simulink model "Neurofeedback_PID_WithoutFNIRS"  (R2021b)
settings: Solver=VariableStepAuto  StartTime=0.0  StopTime=90  FixedStep=0.09  RelTol=1e-8
libraries: slpidlib x1
settings Model: SnapshotInterval=100  Creator=mdls3  LastModifiedBy=mdls3
settings SolverCC: ZeroCrossControl=EnableAll
settings DebuggingCC: UnderSpecifiedDimensionMsg=warning

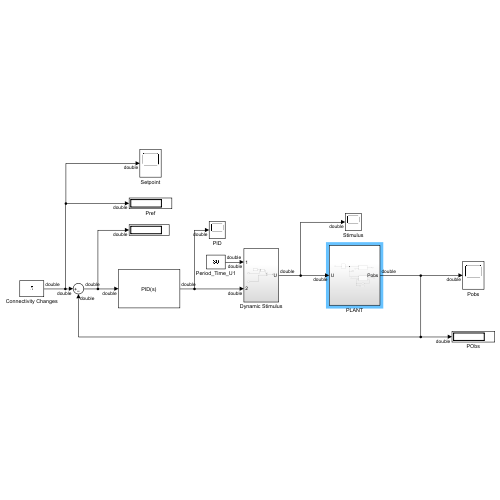
[thumbnail: Simulink's stored preview of the top-level diagram]
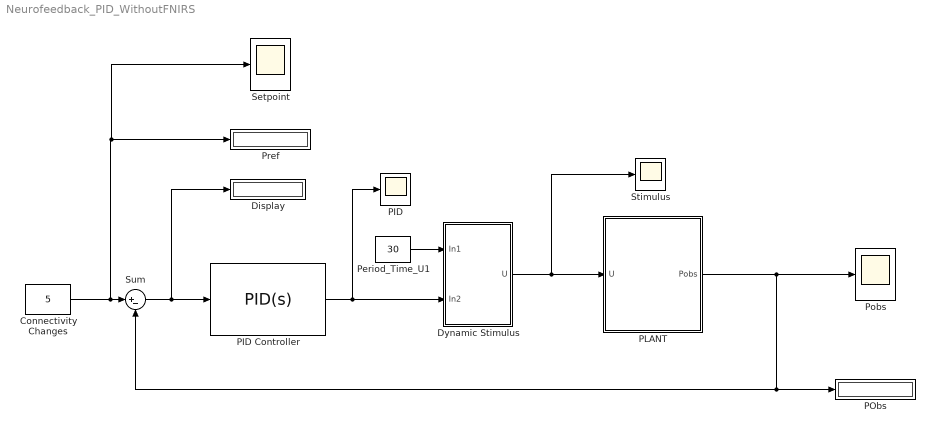
== system Neurofeedback_PID_WithoutFNIRS ==
  Connectivity Changes : Constant  Value=5
  Display : Display
  Dynamic Stimulus : Subsystem
  PID : Scope
  PID Controller : slpidlib/PID Controller  Controller=PID  Form=Ideal  TimeDomain=Continuous-time  UseExternalTs=off  SampleTime=-1  IntegratorMethod=Forward Euler  FilterMethod=Forward Euler  ControllerParametersSource=internal  P=0.2  I=0.1525  D=0.105  UseFilter=on  N=100  TunerSelectOption=Transfer Function Based (PID Tuner App)  InitialConditionSource=internal  InitialConditionForIntegrator=1  InitialConditionForFilter=0  DifferentiatorICPrevScaledInput=0  ExternalReset=none  TrackingMode=off  Kt=1  LimitOutput=off  SatLimitsSource=internal  UpperSaturationLimit=inf  LowerSaturationLimit=-inf  LinearizeAsGain=on  AntiWindupMode=none  Kb=1  POutMin=[]  POutMax=[]  IOutMin=[]  IOutMax=[]  DOutMin=[]  DOutMax=[]  NOutMin=[]  NOutMax=[]  SumOutMin=[]  SumOutMax=[]  SaturationOutMin=[]  SaturationOutMax=[]  PParamMin=[]  PParamMax=[]  IParamMin=[]  IParamMax=[]  DParamMin=[]  DParamMax=[]  NParamMin=[]  NParamMax=[]  KbParamMin=[]  KbParamMax=[]  KtParamMin=[]  KtParamMax=[]  KbOutMin=[]  KbOutMax=[]  KtOutMin=[]  KtOutMax=[]  IntegratorOutMin=[]  IntegratorOutMax=[]  FilterOutMin=[]  FilterOutMax=[]  SumI1OutMin=[]  SumI1OutMax=[]  SumI2OutMin=[]  SumI2OutMax=[]  SumI3OutMin=[]  SumI3OutMax=[]  SumI4OutMin=[]  SumI4OutMax=[]  SumDOutMin=[]  SumDOutMax=[]  DifferentiatorOutMin=[]  DifferentiatorOutMax=[]  FilterDiffOutCoefMin=[]  FilterDiffOutCoefMax=[]  ReciprocalOutMin=[]  ReciprocalOutMax=[]  SumDenOutMin=[]  SumDenOutMax=[]  SumNumOutMin=[]  SumNumOutMax=[]  DivideOutMin=[]  DivideOutMax=[]  UdiffTsProdOutMin=[]  UdiffTsProdOutMax=[]  NTsProdOutMin=[]  NTsProdOutMax=[]  UintegralTsProdOutMin=[]  UintegralTsProdOutMax=[]  UngainTsProdOutMin=[]  UngainTsProdOutMax=[]  IntegratorContinuousStateAttributes=''  IntegratorStateMustResolveToSignalObject=off  IntegratorRTWStateStorageClass=Auto  FilterContinuousStateAttributes=''  FilterStateMustResolveToSignalObject=off  FilterRTWStateStorageClass=Auto  ParallelPVariant=Passthrough  IdealPVariant=InternalParameters  IVariant=InternalParameters  DVariant=InternalParameters  IntegratorVariant=Continuous  SatVariant=Disabled  AWVariant=Passthrough  PCopyVariant=Disabled  TRVariant=Disabled  FdbkBlocksVariant=Forward  IdealPFdbkVariant=Disabled  SatFdbkVariant=Disabled  DerivativeFilterVariant=ContFilter  NVariant=InternalParameters  NCopyVariant=Disabled  FilterICVariant=InternalICsFilter  IntegratorICVariant=InternalICs  ExternalResetVariant=Disabled  TRSumVariant=Passthrough  SumFdbkVariant=Disabled  SumVariant=Sum_PID  TsampFilterVariant=InternalTs  TsampNgainVariant=Passthrough  TsampIntegralVariant=Passthrough  ExternalSaturationOutDataTypeStr=Inherit: Same as second input
  PLANT : Subsystem
  PObs : Display
  Period_Time_U1 : Constant  Value=30
  Pobs : Scope
  Pref : Display
  Setpoint : Scope
  Stimulus : Scope
  Sum : Sum  Inputs=|+-
  wires:
  Period_Time_U1/1 -> Dynamic Stimulus/1(In1)
  Dynamic Stimulus/1(U) -> Stimulus/1, PLANT/1(U)
  PID Controller/1 -> Dynamic Stimulus/2(In2), PID/1
  Sum/1 -> PID Controller/1, Display/1
  Connectivity Changes/1 -> Setpoint/1, Pref/1, Sum/1
  PLANT/1(Pobs) -> Sum/2, PObs/1, Pobs/1

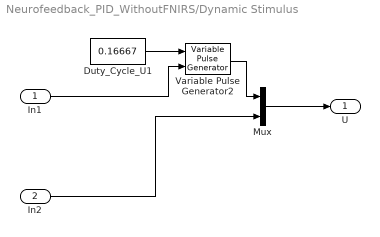
== system Neurofeedback_PID_WithoutFNIRS/Dynamic Stimulus ==
  In1 : Inport
  In2 : Inport  Port=2
  Duty_Cycle_U1 : Constant  Value=0.16667  OutMin=[0]  OutMax=[0.8]
  Mux : Mux  Inputs=2
  Variable Pulse Generator2 : VariablePulseGenerator  RunAtFixedTimeIntervals=on  SampleTime=1/10.4
  U : Outport
  wires:
  In1/1 -> Variable Pulse Generator2/2
  Mux/1 -> U/1
  Variable Pulse Generator2/1 -> Mux/1
  Duty_Cycle_U1/1 -> Variable Pulse Generator2/1
  In2/1 -> Mux/2

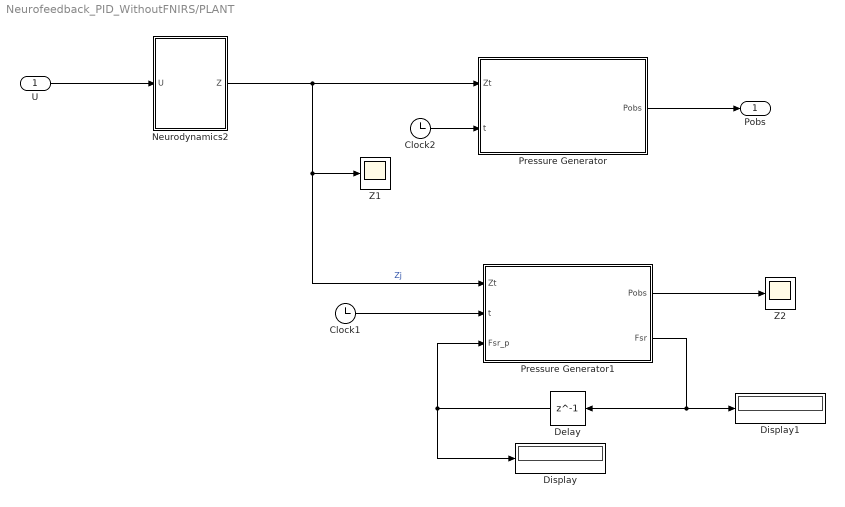
== system Neurofeedback_PID_WithoutFNIRS/PLANT ==
  U : Inport
  Clock1 : Clock
  Clock2 : Clock
  Delay : Delay  DelayLength=1  InitialCondition=0.0001
  Display : Display
  Display1 : Display
  Neurodynamics2 : Subsystem
  Pressure Generator : MATLAB Function  TreatAsAtomicUnit=on
  Pressure Generator1 : MATLAB Function  TreatAsAtomicUnit=on
  Z1 : Scope
  Z2 : Scope
  Pobs : Outport
  wires:
  U/1 -> Neurodynamics2/1(U)
  Neurodynamics2/1(Z) -> Pressure Generator/1(Zt), Pressure Generator1/1(Zt), Z1/1  "Zj"
  Delay/1 -> Display/1, Pressure Generator1/3(Fsr_p)
  Clock1/1 -> Pressure Generator1/2(t)
  Pressure Generator1/2(Fsr) -> Delay/1, Display1/1
  Pressure Generator1/1(Pobs) -> Z2/1
  Clock2/1 -> Pressure Generator/2(t)
  Pressure Generator/1(Pobs) -> Pobs/1

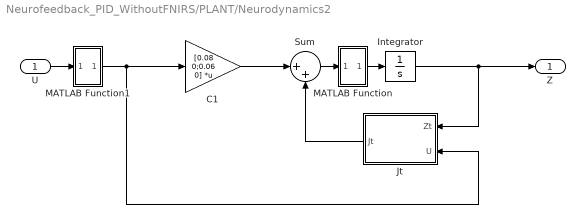
== system Neurofeedback_PID_WithoutFNIRS/PLANT/Neurodynamics2 ==
  U : Inport
  C1 : Gain  Gain=[0.08 0;0.06 0]  Multiplication=Matrix(K*u) (u vector)
  Integrator : Integrator
  Jt : MATLAB Function  TreatAsAtomicUnit=on
  MATLAB Function : MATLAB Function  TreatAsAtomicUnit=on
  MATLAB Function1 : MATLAB Function  TreatAsAtomicUnit=on
  Sum : Sum  Inputs=|++
  Z : Outport
  wires:
  Integrator/1 -> Z/1, Jt/1(Zt)
  C1/1 -> Sum/1
  Jt/1(Jt) -> Sum/2
  U/1 -> MATLAB Function1/1(Z)
  Sum/1 -> MATLAB Function/1(Z)
  MATLAB Function1/1(Zn) -> C1/1, Jt/2(U)
  MATLAB Function/1(Zn) -> Integrator/1

== matlab function Neurofeedback_PID_WithoutFNIRS/PLANT/Pressure Generator ==
  data: Zt input; Pobs output; t input
function Pobs = fcn(Zt, t)
    R=28.2; %Resistor [Ohms];
    C=0.8; %Capacitor [Faradays];
    V= Zt(1,:); %Voltage or system reference;
    Vc = V * (1 - exp(-t/(R*C))); % Voltage at the capacitor  
    
Pobs = Vc;

== matlab function Neurofeedback_PID_WithoutFNIRS/PLANT/Pressure Generator1 ==
  data: Zt input; Pobs output; t input; Fsr_p input; Fsr output
function [Pobs,Fsr] = PressureGenerator_sensor(Zt, t,Fsr_p)
    C = 0.000001; % 0.1uF
    Vcc = 500; %Considering 5V as a real sensor, the value is on mV
    Rf = 10000; %Fixed resistor 10k ohms
    kgf = 0.1019716213; % 1N = 0.1019716213 kgf
    Fsr = 0;
    Fsrforce = 0;

    Vout = Zt(1) * (1 - exp( -t / C)); %Emulation of the capacitor
    Fsr = (Vcc - Vout * Rf) / Vout;
    FsConductance = 1000000; %Sensor conductance in uOhms
    FsConductance = FsConductance / Fsr;
    if FsConductance <= 1000
        Fsrforce = FsConductance / 80; %Force on Newtons
    else
        Fsrforce = FsConductance - 1000;
        Fsrforce = Fsrforce / 30;
    end
    
Pobs = Fsrforce* kgf;

end

== matlab function Neurofeedback_PID_WithoutFNIRS/PLANT/Neurodynamics2/MATLAB Function1 ==
  data: Z input; Zn output
function Zn = fcn(Z)

Zn = Z(:,1);

== matlab function Neurofeedback_PID_WithoutFNIRS/PLANT/Neurodynamics2/MATLAB Function ==
  data: Z input; Zn output
function Zn = fcn(Z)

Zn = Z(:,1);

== matlab function Neurofeedback_PID_WithoutFNIRS/PLANT/Neurodynamics2/Jt ==
  data: Zt input; U input; Jt output
function Jt = fcn(Zt, U)
   A = [-0.16 -0.49;-0.02 -0.33];
   nRegions  = size(A,1);
   M = size(U,1); %nStimuli
   simulationLength = size(U,2);
   B = zeros(2,2,2);
   B1 = [0 0; 0 0]; %There must be a B per stimulus
   %B2 = [-0.02 -0.77; 0.33 -1.31];
   B2 = [-0.1103 0.4004; 0.8658 -1.431];
   B(:,:,1) = B1;
   B(:,:,2) = B2;
      assert(M == size(B,3),...
       'Unexpected number of induced connectivity parameters B.');
   T = zeros(nRegions); %nRegions x nRegions
    for t = 1:simulationLength
           for uu = 1:M % Sum (Uj * Bj)
               tmp = U(uu,t)*B(:,:,uu);
               T = -0.5*exp(T + tmp);  
           end
    end
    SI = diag(A);
    A =  A - diag(exp(SI) + (SI));
Jt = (A*Zt) + (T*Zt);
